simulink model "ConditionAction_2018a"  (R2018a)
settings: Solver=VariableStepAuto  StartTime=0.0  StopTime=10.0  RelTol=1e-3
settings Model: Creator=apple  LastModifiedBy=apple
settings DataIOCC: ReturnWorkspaceOutputs=on
settings SFSimCC: SimUseLocalCustomCode=on
settings RTWCC: RTWUseLocalCustomCode=on

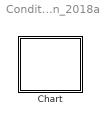
== system ConditionAction_2018a ==
  Chart : Stateflow chart  TreatAsAtomicUnit=on

== stateflow chart ConditionAction_2018a/Chart ==
  state C
    en:fprintf("Entry C");
    du:fprintf("During C");
    ex:fprintf("Exit C");
  state A
    en:fprintf("Entry A");
    du:fprintf("During A");
    ex:fprintf("Exit A");
  state B
    en:fprintf("Entry B");
    du:fprintf("During B");
    ex:fprintf("Exit B");
  (default) -> A : {x = 0;}
  A -> (junction 5) : E_one{fprintf("Condition Action1")}
  (junction 5) -> C [order 1] : [x>0]
  (junction 5) -> B [order 2]
  data: x local
  events: E_one local FUNCTION_CALL_EVENT
